simulink model "Ito"  (R2022b)
settings: Solver=VariableStepAuto  StartTime=0.0  StopTime=2000  RelTol=1e-3
values from neighbouring files (symbols this model uses):
  EK = (R*T)/F*log(Ko / Ki)    [RunMe.m]
  GtoSlow = 0.0376    [RunMe.m]
  Vm = Vm_values(i)    [RunMe.m]
settings Model: Creator=Utente  LastModifiedBy=Utente

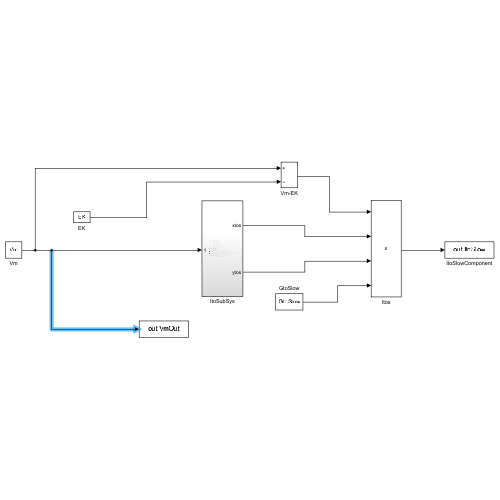
[thumbnail: Simulink's stored preview of the top-level diagram]
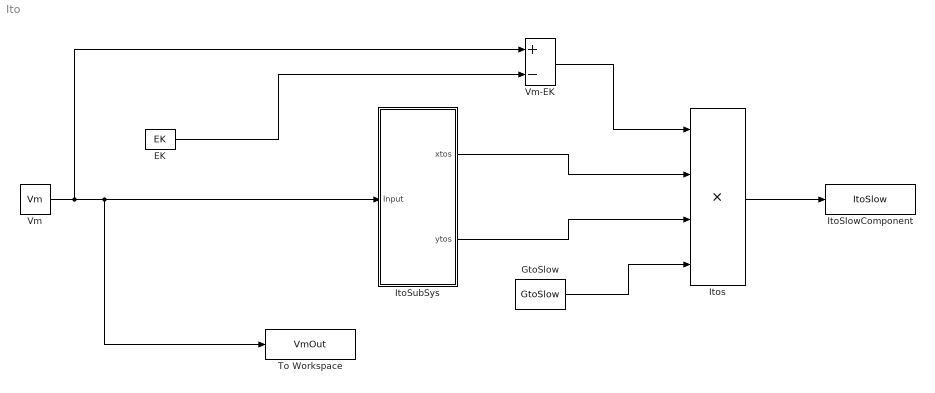
== system Ito ==
  EK : Constant  Value=EK
  GtoSlow : Constant  Value=GtoSlow
  ItoSlowComponent : ToWorkspace  VariableName=ItoSlow  SampleTime=-1
  ItoSubSys : Subsystem
  Itos : Product  Inputs=4
  To Workspace : ToWorkspace  VariableName=VmOut  SampleTime=-1
  Vm : Constant  Value=Vm
  Vm-EK : Sum  Inputs=+-
  wires:
  Vm/1 -> Vm-EK/1, To Workspace/1, ItoSubSys/1(Input)
  ItoSubSys/2(ytos) -> Itos/3
  EK/1 -> Vm-EK/2
  Itos/1 -> ItoSlowComponent/1
  ItoSubSys/1(xtos) -> Itos/2
  Vm-EK/1 -> Itos/1
  GtoSlow/1 -> Itos/4

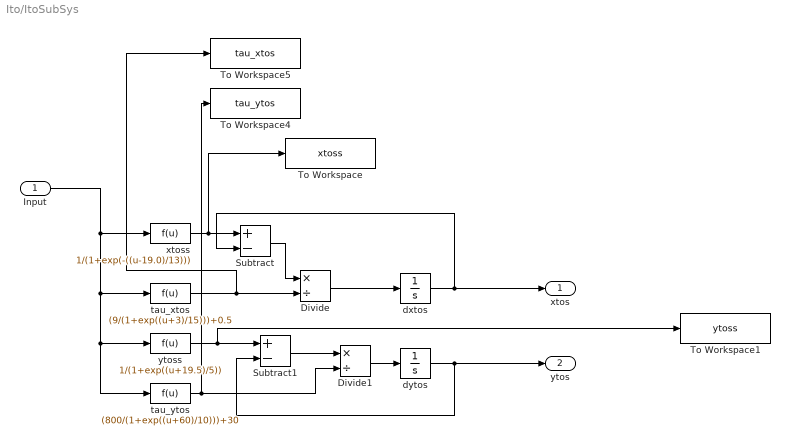
== system Ito/ItoSubSys ==
  Input : Inport
  " dxtos" : Integrator
  Divide : Product  Inputs=*/
  Divide1 : Product  Inputs=*/
  Subtract : Sum  Inputs=+-
  Subtract1 : Sum  Inputs=+-
  To Workspace : ToWorkspace  VariableName=xtoss  SampleTime=-1
  To Workspace1 : ToWorkspace  VariableName=ytoss  SampleTime=-1
  To Workspace4 : ToWorkspace  VariableName=tau_ytos  SampleTime=-1
  To Workspace5 : ToWorkspace  VariableName=tau_xtos  SampleTime=-1
  dytos : Integrator  InitialCondition=1
  tau_xtos : Fcn  Expr=(9/(1+exp((u+3)/15)))+0.5
  tau_ytos : Fcn  Expr=(800/(1+exp((u+60)/10)))+30
  xtoss : Fcn  Expr=1/(1+exp(-((u-19.0)/13)))
  ytoss : Fcn  Expr=1/(1+exp((u+19.5)/5))
  xtos : Outport
  ytos : Outport  Port=2
  wires:
  ytoss/1 -> To Workspace1/1, Subtract1/1
  Input/1 -> tau_ytos/1, ytoss/1, tau_xtos/1, xtoss/1
  Divide1/1 -> dytos/1
  " dxtos"/1 -> xtos/1, Subtract/2
  tau_ytos/1 -> To Workspace4/1, Divide1/2
  dytos/1 -> ytos/1, Subtract1/2
  tau_xtos/1 -> To Workspace5/1, Divide/2
  Divide/1 -> " dxtos"/1
  Subtract/1 -> Divide/1
  Subtract1/1 -> Divide1/1
  xtoss/1 -> To Workspace/1, Subtract/1
